simulink model "untitled"  (R2021b)
settings: Solver=FixedStepDiscrete  StartTime=0.0  StopTime=inf  FixedStep=0.0005  RelTol=1e-3
undefined symbols (not defined in the file or in its folder): f
libraries: instrumentlib x2, dspfdesign x1
settings Model: Creator=Administrator  LastModifiedBy=frekle
settings SolverCC: AlgebraicLoopSolver=TrustRegion
settings DebuggingCC: SFMachineParentedDataDiag=warning

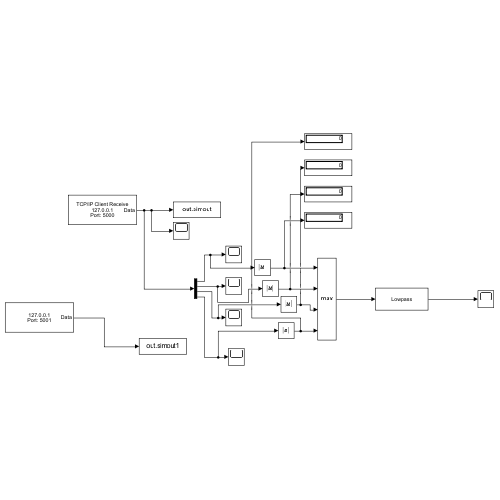
[thumbnail: Simulink's stored preview of the top-level diagram]
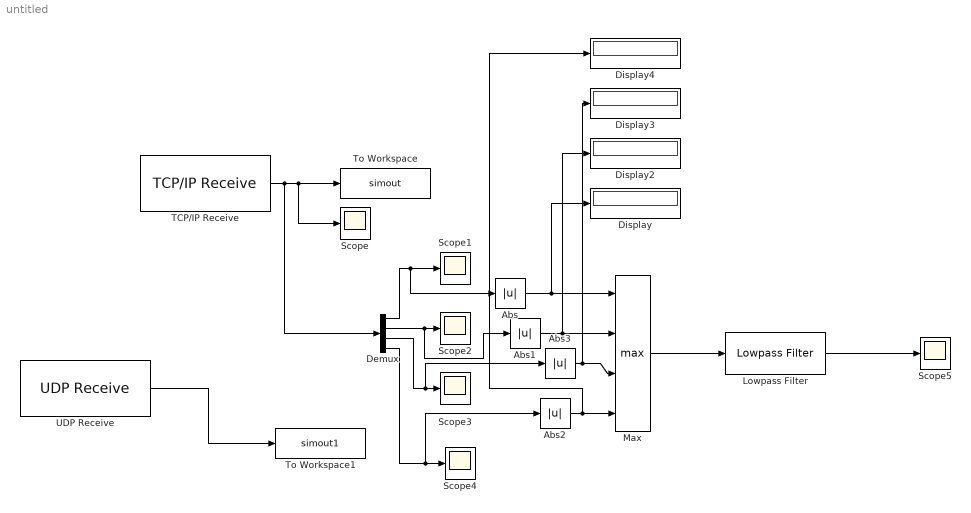
== system untitled ==
  Abs{,1..3} (4 alike) : Abs
  Demux : Demux
  Display{,2..4} (4 alike) : Display
  Lowpass Filter : dspfdesign/Lowpass Filter  FilterType=FIR  DesignForMinimumOrder=off  FilterOrder=4  PassbandFrequency=20  StopbandFrequency=12e3  PassbandRipple=0.1  StopbandAttenuation=80  InheritSampleRate=off  SampleRate=2000  SimulateUsing=Interpreted execution  roundingMode=Floor  coeffsDataTypeStr=fixdt(1,16)
  Max : MinMax  Function=max  Inputs=4
  Scope{,1..5} (6 alike) : Scope
  TCP/IP Receive : instrumentlib/TCP//IP Receive  Host=127.0.0.1  Port=5000  DataSize=320  DataType=double  ASCIIFormatting=%f%f%f%f,  Terminator=LF  CustomTerminator=10  ByteOrder=little-endian  EnableBlockingMode=on  Timeout=10  SampleTime=0.0005  SimulateUsing=Interpreted execution
  To Workspace : ToWorkspace  VariableName=simout  SaveFormat=Timeseries  SampleTime=-1
  To Workspace1 : ToWorkspace  VariableName=simout1  SaveFormat=Timeseries  SampleTime=-1
  UDP Receive : instrumentlib/UDP Receive  Host=localhost  Port=9090  LocalPort=5001  EnablePortSharing=off  GetLatestData=off  DataSize=320  DataType=double  ASCIIFormatting=%f,  Terminator=LF  ByteOrder=LittleEndian  EnableBlockingMode=on  Timeout=10  SampleTime=0.01  LocalAddress=127.0.0.1
  wires:
  TCP/IP Receive/1 -> Demux/1, Scope/1, To Workspace/1
  Demux/1 -> Abs/1, Scope1/1
  Demux/2 -> Abs1/1, Scope2/1
  Demux/4 -> Abs2/1, Scope4/1
  Demux/3 -> Abs3/1, Scope3/1
  Abs/1 -> Display/1, Max/1
  Abs1/1 -> Display2/1, Max/2
  Abs3/1 -> Display3/1, Max/3
  Abs2/1 -> Display4/1, Max/4
  Max/1 -> Lowpass Filter/1
  Lowpass Filter/1 -> Scope5/1
  UDP Receive/1 -> To Workspace1/1
